simulink model "Backup_of_FOC_Simulate"  (R2016b)
settings: Solver=ode1  StartTime=0.0  StopTime=20  FixedStep=1e-5  RelTol=1e-3  EnableMultiTasking=on
undefined symbols (not defined in the file): sigbuilder_block
libraries: simulink x9, powerlib_meascontrol x4, powerlib x4
settings Model: ExtModeTrigDuration=8  Creator=tiend  LastModifiedBy=tiend

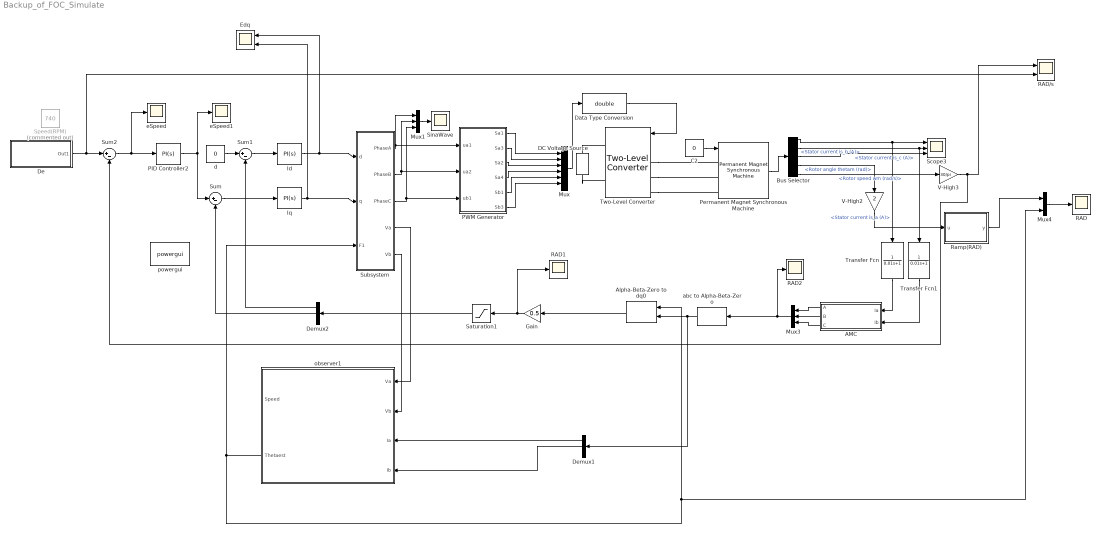
== system Backup_of_FOC_Simulate ==
  AMC : Subsystem
  Alpha-Beta-Zero to dq0 : powerlib_meascontrol/Transformations/Alpha-Beta-Zero to dq0  Alignment=Aligned with phase A axis
  Bus Selector : BusSelector  OutputSignals=Stator current is_a (A),Stator current is_b (A),Stator current is_c (A),Rotor angle thetam (rad),Rotor speed wm (rad/s)
  C2 : Constant  Value=0
  DC Voltage Source : powerlib/Electrical Sources/DC Voltage Source  Amplitude=300  Measurements=Voltage
  Data Type Conversion : DataTypeConversion  OutDataTypeStr=double
  De : Subsystem
  Demux1 : Demux  Outputs=3
  Demux2 : Demux  Outputs=3
  Edq : Scope  NumInputPorts=2
  Gain : Gain  Gain=0.5
  Id : simulink/Continuous/PID Controller  Controller=PI  TimeDomain=Continuous-time  SampleTime=-1  IntegratorMethod=Forward Euler  FilterMethod=Forward Euler  Form=Parallel  UseFilter=on  ControllerParametersSource=internal  P=0.5  I=0.5  D=0  N=100  InitialConditionSource=internal  InitialConditionForIntegrator=0  InitialConditionForFilter=0  ExternalReset=none  LimitOutput=off  UpperSaturationLimit=inf  LowerSaturationLimit=-inf  LinearizeAsGain=on  AntiWindupMode=none  Kb=1  TrackingMode=off  Kt=1  PParamMin=[]  PParamMax=[]  IParamMin=[]  IParamMax=[]  DParamMin=[]  DParamMax=[]  NParamMin=[]  NParamMax=[]  KbParamMin=[]  KbParamMax=[]  KtParamMin=[]  KtParamMax=[]  POutMin=[]  POutMax=[]  IOutMin=[]  IOutMax=[]  DOutMin=[]  DOutMax=[]  NOutMin=[]  NOutMax=[]  KbOutMin=[]  KbOutMax=[]  KtOutMin=[]  KtOutMax=[]  IntegratorOutMin=[]  IntegratorOutMax=[]  FilterOutMin=[]  FilterOutMax=[]  SumOutMin=[]  SumOutMax=[]  SumI1OutMin=[]  SumI1OutMax=[]  SumI2OutMin=[]  SumI2OutMax=[]  SumI3OutMin=[]  SumI3OutMax=[]  SumDOutMin=[]  SumDOutMax=[]  SaturationOutMin=[]  SaturationOutMax=[]  IntegratorContinuousStateAttributes=''  IntegratorStateMustResolveToSignalObject=off  IntegratorRTWStateStorageClass=Auto  FilterContinuousStateAttributes=''  FilterStateMustResolveToSignalObject=off  FilterRTWStateStorageClass=Auto  DifferentiatorICPrevScaledInput=0  DifferentiatorOutMin=[]  DifferentiatorOutMax=[]
  Iq : simulink/Continuous/PID Controller  Controller=PI  TimeDomain=Continuous-time  SampleTime=-1  IntegratorMethod=Forward Euler  FilterMethod=Forward Euler  Form=Parallel  UseFilter=on  ControllerParametersSource=internal  P=0.7  I=0.9  D=0  N=100  InitialConditionSource=internal  InitialConditionForIntegrator=0  InitialConditionForFilter=0  ExternalReset=none  LimitOutput=off  UpperSaturationLimit=inf  LowerSaturationLimit=-inf  LinearizeAsGain=on  AntiWindupMode=none  Kb=1  TrackingMode=off  Kt=1  PParamMin=[]  PParamMax=[]  IParamMin=[]  IParamMax=[]  DParamMin=[]  DParamMax=[]  NParamMin=[]  NParamMax=[]  KbParamMin=[]  KbParamMax=[]  KtParamMin=[]  KtParamMax=[]  POutMin=[]  POutMax=[]  IOutMin=[]  IOutMax=[]  DOutMin=[]  DOutMax=[]  NOutMin=[]  NOutMax=[]  KbOutMin=[]  KbOutMax=[]  KtOutMin=[]  KtOutMax=[]  IntegratorOutMin=[]  IntegratorOutMax=[]  FilterOutMin=[]  FilterOutMax=[]  SumOutMin=[]  SumOutMax=[]  SumI1OutMin=[]  SumI1OutMax=[]  SumI2OutMin=[]  SumI2OutMax=[]  SumI3OutMin=[]  SumI3OutMax=[]  SumDOutMin=[]  SumDOutMax=[]  SaturationOutMin=[]  SaturationOutMax=[]  IntegratorContinuousStateAttributes=''  IntegratorStateMustResolveToSignalObject=off  IntegratorRTWStateStorageClass=Auto  FilterContinuousStateAttributes=''  FilterStateMustResolveToSignalObject=off  FilterRTWStateStorageClass=Auto  DifferentiatorICPrevScaledInput=0  DifferentiatorOutMin=[]  DifferentiatorOutMax=[]
  Mux : Mux  Inputs=6
  Mux1 : Mux  Inputs=3
  Mux3 : Mux  Inputs=3
  Mux4 : Mux  Inputs=2
  PID Controller2 : simulink/Continuous/PID Controller  Controller=PI  TimeDomain=Continuous-time  SampleTime=-1  IntegratorMethod=Forward Euler  FilterMethod=Forward Euler  Form=Parallel  UseFilter=on  ControllerParametersSource=internal  P=1/50  I=0.01  D=0  N=100  InitialConditionSource=internal  InitialConditionForIntegrator=0  InitialConditionForFilter=0  ExternalReset=none  LimitOutput=off  UpperSaturationLimit=1  LowerSaturationLimit=-0.1  LinearizeAsGain=on  AntiWindupMode=none  Kb=1  TrackingMode=off  Kt=1  PParamMin=[]  PParamMax=[]  IParamMin=[]  IParamMax=[]  DParamMin=[]  DParamMax=[]  NParamMin=[]  NParamMax=[]  KbParamMin=[]  KbParamMax=[]  KtParamMin=[]  KtParamMax=[]  POutMin=[]  POutMax=[]  IOutMin=[]  IOutMax=[]  DOutMin=[]  DOutMax=[]  NOutMin=[]  NOutMax=[]  KbOutMin=[]  KbOutMax=[]  KtOutMin=[]  KtOutMax=[]  IntegratorOutMin=[]  IntegratorOutMax=[]  FilterOutMin=[]  FilterOutMax=[]  SumOutMin=[]  SumOutMax=[]  SumI1OutMin=[]  SumI1OutMax=[]  SumI2OutMin=[]  SumI2OutMax=[]  SumI3OutMin=[]  SumI3OutMax=[]  SumDOutMin=[]  SumDOutMax=[]  SaturationOutMin=[]  SaturationOutMax=[]  IntegratorContinuousStateAttributes=''  IntegratorStateMustResolveToSignalObject=off  IntegratorRTWStateStorageClass=Auto  FilterContinuousStateAttributes=''  FilterStateMustResolveToSignalObject=off  FilterRTWStateStorageClass=Auto  DifferentiatorICPrevScaledInput=0  DifferentiatorOutMin=[]  DifferentiatorOutMax=[]
  PWM Generator : Subsystem
  Permanent Magnet Synchronous Machine : powerlib/Machines/Permanent Magnet Synchronous Machine  NbPhases=3  FluxDistribution=Sinusoidal  RotorType=Round  MechanicalLoad=Torque Tm  PresetModel="01:  0.8 Nm 300 Vdc 3000 RPM - 0.8 Nm"  ShowDetailedParameters=on  MeasurementBus=off  Resistance=18.7  Inductance=8.5e-3  dqInductances=[8.5e-3,8.5e-3]  La=0.02682  MachineConstant=Flux linkage established by magnets (V.s)  Flux=0.1717  VoltageCst=62.2859  TorqueCst=0.5151  Flat=120  Mechanical=[2.26e-05 1.349e-05 2 0]  PolePairs=2  InitialConditions=[0,30, 0,0]  InitialConditions5ph=[0 0 0 0 0 0]  TsPowergui=0  TsBlock=-1  RefAngle=Aligned with phase A axis (original Park)
  RAD : Scope
  RAD/s : Scope  NumInputPorts=2
  RAD1 : Scope
  RAD2 : Scope
  Ramp(RAD) : MATLAB Function  TreatAsAtomicUnit=on
  Saturation1 : Saturate  UpperLimit=1  LowerLimit=-1
  Scope3 : Scope  NumInputPorts=3
  SinaWave : Scope
  Speed(RPM) : Constant  Commented=on  Value=740
  Subsystem : Subsystem
  Sum : Sum  Inputs=|+-
  Sum1 : Sum  Inputs=|+-
  Sum2 : Sum  Inputs=|+-
  Transfer Fcn : TransferFcn  Denominator=[0.01 1]
  Transfer Fcn1 : TransferFcn  Denominator=[0.01 1]
  Two-Level Converter : powerlib/Power Electronics/Two-Level Converter  ModelType=Switching devices  Ron=1e-3  Rs=1e6  Cs=inf  Vforward=[0,0]  Ron_Diode=1e-3  Rs_Diode=1e6  Cs_Diode=inf  Vf_Diode=1e-3  Rs_CurrentSource=inf
  V-High2 : Gain  Gain=2
  V-High3 : Gain  Gain=30/pi
  abc to Alpha-Beta-Zero : powerlib_meascontrol/Transformations/abc to Alpha-Beta-Zero
  d : Constant  Value=0
  eSpeed : Scope
  eSpeed1 : Scope
  observer1 : Subsystem  mask{R=0.0485, L=0.000395, Pva=20, Iva=0.1, Pvb=20, Ivb=0.1, K1=10, K2=5}
  powergui : powerlib/powergui  Priority=1  SimulationMode=Discrete  SolverType=Tustin/Backward Euler (TBE)  SampleTime=1e-5  frequency=60  SPID=off  DisableSnubberDevices=off  DisableRonSwitches=off  DisableVfSwitches=off  SwTol=0  DisplayEquations=off  Interpol=off  ExternalGateDelay=off  methode=off  Ts=10  FunctionMessages=off  echomessages=off  HookPort=off  EnableUseOfTLC=off  x0status=blocks  frequencyindice=0  Pbase=100e6  ErrMax=1e-4  Iterations=50  UnitsV=kV  UnitsW=MW  buscounter=0  RestoreLinks=warning  ResistiveCurrentMeasurement=off  Frange=[0:2:500]  Ylog=off  Xlog=on  ShowGrid=off  save=off  variable=ZData  structure=0  ZoomFFT=off  StartTime=0.0  cycles=1  DisplayStyle=1  fundamental=60  FreqAxis=off  MaxFrequency=1000  frequencyindicesteady=1  RmsSteady=1  display=off
  wires:
  Subsystem/3(PhaseC) -> PWM Generator/3(ub1), Mux1/3
  Subsystem/2(PhaseB) -> PWM Generator/2(ua2), Mux1/2
  PWM Generator/3(Sa2) -> Mux/3
  PWM Generator/4(Sa4) -> Mux/4
  PWM Generator/2(Sa3) -> Mux/2
  PWM Generator/5(Sb1) -> Mux/5
  PWM Generator/1(Sa1) -> Mux/1
  PWM Generator/6(Sb3) -> Mux/6
  C2/1 -> Permanent Magnet Synchronous Machine/1
  Mux/1 -> Data Type Conversion/1
  Data Type Conversion/1 -> Two-Level Converter/1
  Permanent Magnet Synchronous Machine/1 -> Bus Selector/1
  Mux1/1 -> SinaWave/1
  Subsystem/1(PhaseA) -> PWM Generator/1(ua1), Mux1/1
  Bus Selector/1 -> Scope3/1, Transfer Fcn/1  "<Stator current is_a (A)>"
  Bus Selector/2 -> Transfer Fcn1/1, Scope3/2  "<Stator current is_b (A)>"
  Bus Selector/3 -> Scope3/3  "<Stator current is_c (A)>"
  Bus Selector/4 -> V-High2/1  "<Rotor angle thetam (rad)>"
  AMC/3(C) -> Mux3/3
  AMC/2(B) -> Mux3/2
  AMC/1(A) -> Mux3/1
  Mux3/1 -> abc to Alpha-Beta-Zero/1, RAD2/1
  V-High2/1 -> Ramp(RAD)/1(u)
  Ramp(RAD)/1(y) -> Mux4/1
  Mux4/1 -> RAD/1
  Bus Selector/5 -> V-High3/1  "<Rotor speed wm (rad/s)>"
  Gain/1 -> Saturation1/1, RAD1/1
  d/1 -> Sum1/1
  Sum1/1 -> Id/1
  Id/1 -> Subsystem/1(d), Edq/1
  Sum2/1 -> PID Controller2/1, eSpeed/1
  PID Controller2/1 -> Sum/1, eSpeed1/1
  Saturation1/1 -> Demux2/1
  Demux2/1 -> Sum1/2
  De/1(Out1) -> RAD/s/2, Sum2/1
  Sum/1 -> Iq/1
  Demux2/2 -> Sum/2
  Iq/1 -> Subsystem/2(q), Edq/2
  Subsystem/5(Vb) -> observer1/2(Vb)
  Subsystem/4(Va) -> observer1/1(Va)
  observer1/2(Thetaest) -> Subsystem/3(F1), Alpha-Beta-Zero to dq0/2, Mux4/2
  abc to Alpha-Beta-Zero/1 -> Demux1/1, Alpha-Beta-Zero to dq0/1
  Alpha-Beta-Zero to dq0/1 -> Gain/1
  Demux1/1 -> observer1/3(Ia)
  Demux1/2 -> observer1/4(Ib)
  Transfer Fcn1/1 -> AMC/2(Ib)
  Transfer Fcn/1 -> AMC/1(Ia)
  V-High3/1 -> Sum2/2, RAD/s/1
  connections:
  Two-Level Converter/LConn1 -- Permanent Magnet Synchronous Machine/LConn1
  Two-Level Converter/LConn2 -- Permanent Magnet Synchronous Machine/LConn2
  Two-Level Converter/LConn3 -- Permanent Magnet Synchronous Machine/LConn3
  DC Voltage Source/RConn1 -- Two-Level Converter/RConn1
  DC Voltage Source/LConn1 -- Two-Level Converter/RConn2

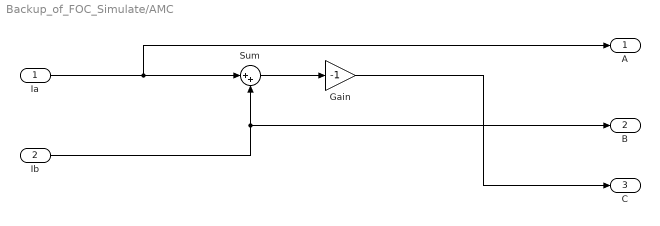
== system Backup_of_FOC_Simulate/AMC ==
  Ia : Inport
  Ib : Inport  Port=2
  Gain : Gain  Gain=-1
  Sum : Sum  Inputs=|++
  A : Outport
  B : Outport  Port=2
  C : Outport  Port=3
  wires:
  Sum/1 -> Gain/1
  Ia/1 -> A/1, Sum/1
  Ib/1 -> B/1, Sum/2
  Gain/1 -> C/1

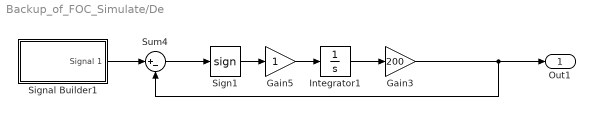
== system Backup_of_FOC_Simulate/De ==
  Gain3 : Gain  Gain=200
  Gain5 : Gain
  Integrator1 : Integrator
  Sign1 : Signum  ZeroCross=off
  Signal Builder1 : Subsystem  Tag=STV Subsys  LoadFcn=sigbuilder_block('load');  StartFcn=sigbuilder_block('start');  StopFcn=sigbuilder_block('stop');  ClipboardFcn=sigbuilder_block('clipboard');  mask(Sigbuilder block){tuvar=[0:10]}
      mask help: Simulink:masks:SigbuilderBlock_MD
      mask init:
      | if ~strcmp(get_param(bdroot(gcbh),'SimulationStatus'),'stopped') tuvar = sigbuilder_block('maskInit'); end
      settings: CopyFcn=sigbuilder_block('copy');  DeleteFcn=sigbuilder_block('delete');  ModelCloseFcn=sigbuilder_block('modelClose');  PreSaveFcn=sigbuilder_block('preSave');  PauseFcn=sigbuilder_block('pause');  ContinueFcn=sigbuilder_block('continue');  NameChangeFcn=sigbuilder_block('namechange');  OpenFcn=sigbuilder_block('open',[437.25 153 550.5 359.25 ]);  CloseFcn=sigbuilder_block('close');
      mask Display: plot(0, 0, 100, 100,[2, 2, 32, 32, 2], [68, 8, 8, 68, 68],[32, 2], [38, 38], [32, 19, 2],[53, 60, 44], [32, 17, 17, 2],[16, 16, 31, 31]);txt = getActiveGroup(gcbh);text(2, 100, txt,'verticalAlignment', 'top');
  Sum4 : Sum  Inputs=|+-
  Out1 : Outport
  wires:
  Signal Builder1/1(Signal 1) -> Sum4/1
  Integrator1/1 -> Gain3/1
  Sum4/1 -> Sign1/1
  Sign1/1 -> Gain5/1
  Gain5/1 -> Integrator1/1
  Gain3/1 -> Out1/1, Sum4/2

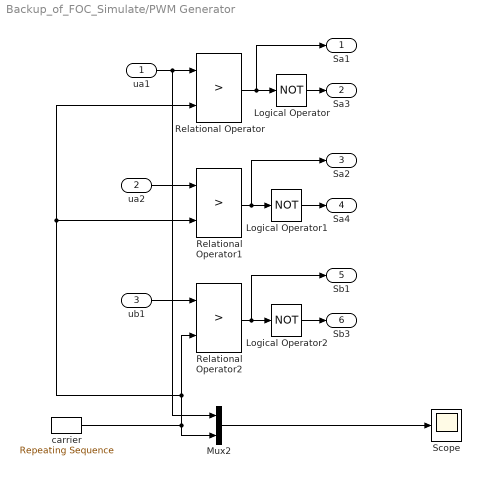
== system Backup_of_FOC_Simulate/PWM Generator ==
  ua1 : Inport
  ua2 : Inport  Port=2
  ub1 : Inport  Port=3
  Logical Operator : Logic  Operator=NOT  AllPortsSameDT=off  OutDataTypeStr=boolean
  Logical Operator1 : Logic  Operator=NOT  AllPortsSameDT=off  OutDataTypeStr=boolean
  Logical Operator2 : Logic  Operator=NOT  AllPortsSameDT=off  OutDataTypeStr=boolean
  Mux2 : Mux  Inputs=2
  Relational Operator : RelationalOperator  Operator=>  OutDataTypeStr=boolean  RndMeth=Nearest
  Relational Operator1 : RelationalOperator  Operator=>  OutDataTypeStr=boolean  RndMeth=Nearest
  Relational Operator2 : RelationalOperator  Operator=>  OutDataTypeStr=boolean  RndMeth=Nearest
  Scope : Scope
  carrier : simulink/Sources/Repeating Sequence  rep_seq_t=[0 1/20000 1/10000]  rep_seq_y=[0 1 0]
  Sa1 : Outport
  Sa3 : Outport  Port=2
  Sa2 : Outport  Port=3
  Sa4 : Outport  Port=4
  Sb1 : Outport  Port=5
  Sb3 : Outport  Port=6
  wires:
  Logical Operator2/1 -> Sb3/1
  Logical Operator1/1 -> Sa4/1
  ub1/1 -> Relational Operator2/1
  ua2/1 -> Relational Operator1/1
  Relational Operator2/1 -> Sb1/1, Logical Operator2/1
  Relational Operator1/1 -> Sa2/1, Logical Operator1/1
  ua1/1 -> Mux2/1, Relational Operator/1
  Relational Operator/1 -> Logical Operator/1, Sa1/1
  Logical Operator/1 -> Sa3/1
  carrier/1 -> Mux2/2, Relational Operator/2, Relational Operator1/2, Relational Operator2/2
  Mux2/1 -> Scope/1

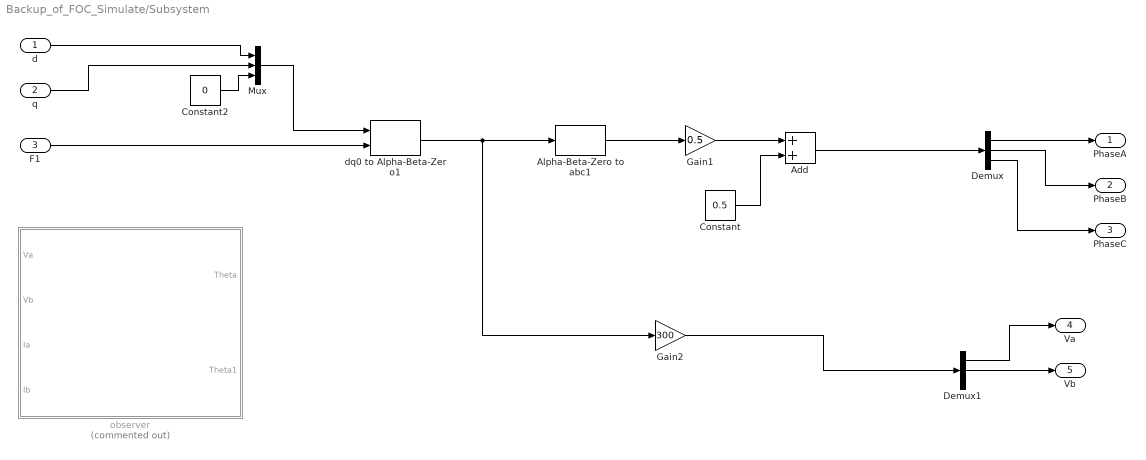
== system Backup_of_FOC_Simulate/Subsystem ==
  d : Inport
  q : Inport  Port=2
  F1 : Inport  Port=3
  Add : Sum
  Alpha-Beta-Zero to abc1 : powerlib_meascontrol/Transformations/Alpha-Beta-Zero to abc
  Constant : Constant  Value=0.5  SampleTime=-1
  Constant2 : Constant  Value=0  SampleTime=-1
  Demux : Demux  Outputs=3
  Demux1 : Demux  Outputs=3
  Gain1 : Gain  Gain=0.5
  Gain2 : Gain  Gain=300
  Mux : Mux  Inputs=3
  dq0 to Alpha-Beta-Zero1 : powerlib_meascontrol/Transformations/dq0 to Alpha-Beta-Zero  Alignment=Aligned with phase A axis
  observer : Subsystem  Commented=on  mask{R=0.0485, L=0.000395, Pva=17, Iva=0.1, Pvb=17, Ivb=0.1, K1=10, K2=5}
  PhaseA : Outport
  PhaseB : Outport  Port=2
  PhaseC : Outport  Port=3
  Va : Outport  Port=4
  Vb : Outport  Port=5
  wires:
  Constant/1 -> Add/2
  Alpha-Beta-Zero to abc1/1 -> Gain1/1
  Demux/1 -> PhaseA/1
  Demux/2 -> PhaseB/1
  Demux/3 -> PhaseC/1
  Mux/1 -> dq0 to Alpha-Beta-Zero1/1
  Add/1 -> Demux/1
  Constant2/1 -> Mux/3
  d/1 -> Mux/1
  Gain1/1 -> Add/1
  F1/1 -> dq0 to Alpha-Beta-Zero1/2
  q/1 -> Mux/2
  dq0 to Alpha-Beta-Zero1/1 -> Gain2/1, Alpha-Beta-Zero to abc1/1
  Demux1/1 -> Va/1
  Demux1/2 -> Vb/1
  Gain2/1 -> Demux1/1

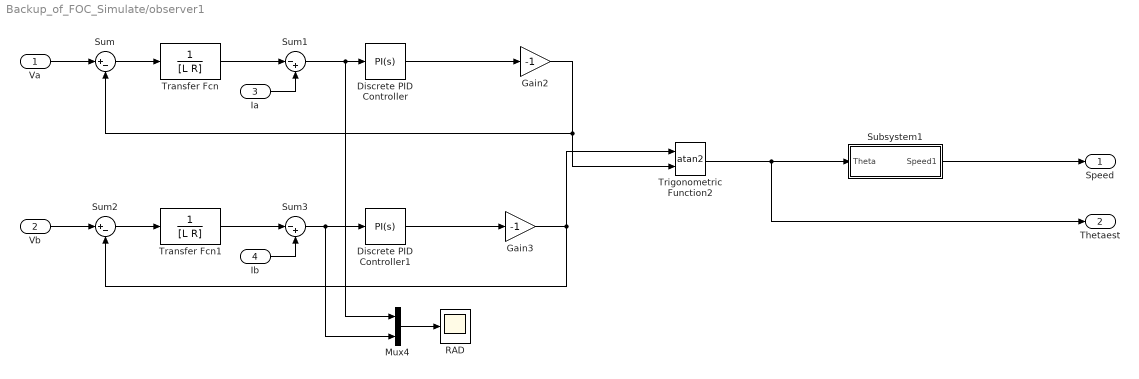
== system Backup_of_FOC_Simulate/observer1 ==
  Va : Inport
  Vb : Inport  Port=2
  Ia : Inport  Port=3
  Ib : Inport  Port=4
  Discrete PID Controller : simulink/Continuous/PID Controller  Controller=PI  TimeDomain=Continuous-time  SampleTime=-1  IntegratorMethod=Forward Euler  FilterMethod=Forward Euler  Form=Parallel  UseFilter=on  ControllerParametersSource=internal  P=Pva  I=Iva  D=0  N=100  InitialConditionSource=internal  InitialConditionForIntegrator=0  InitialConditionForFilter=0  ExternalReset=none  LimitOutput=off  UpperSaturationLimit=inf  LowerSaturationLimit=-inf  LinearizeAsGain=off  AntiWindupMode=none  Kb=1  TrackingMode=off  Kt=1  PParamMin=[]  PParamMax=[]  IParamMin=[]  IParamMax=[]  DParamMin=[]  DParamMax=[]  NParamMin=[]  NParamMax=[]  KbParamMin=[]  KbParamMax=[]  KtParamMin=[]  KtParamMax=[]  POutMin=[]  POutMax=[]  IOutMin=[]  IOutMax=[]  DOutMin=[]  DOutMax=[]  NOutMin=[]  NOutMax=[]  KbOutMin=[]  KbOutMax=[]  KtOutMin=[]  KtOutMax=[]  IntegratorOutMin=[]  IntegratorOutMax=[]  FilterOutMin=[]  FilterOutMax=[]  SumOutMin=[]  SumOutMax=[]  SumI1OutMin=[]  SumI1OutMax=[]  SumI2OutMin=[]  SumI2OutMax=[]  SumI3OutMin=[]  SumI3OutMax=[]  SumDOutMin=[]  SumDOutMax=[]  SaturationOutMin=[]  SaturationOutMax=[]  IntegratorContinuousStateAttributes=''  IntegratorStateMustResolveToSignalObject=off  IntegratorRTWStateStorageClass=Auto  FilterContinuousStateAttributes=''  FilterStateMustResolveToSignalObject=off  FilterRTWStateStorageClass=Auto  DifferentiatorICPrevScaledInput=0  DifferentiatorOutMin=[]  DifferentiatorOutMax=[]
  Discrete PID Controller1 : simulink/Continuous/PID Controller  Controller=PI  TimeDomain=Continuous-time  SampleTime=-1  IntegratorMethod=Forward Euler  FilterMethod=Forward Euler  Form=Parallel  UseFilter=on  ControllerParametersSource=internal  P=Pvb  I=Ivb  D=0  N=100  InitialConditionSource=internal  InitialConditionForIntegrator=0  InitialConditionForFilter=0  ExternalReset=none  LimitOutput=off  UpperSaturationLimit=inf  LowerSaturationLimit=-inf  LinearizeAsGain=off  AntiWindupMode=none  Kb=1  TrackingMode=off  Kt=1  PParamMin=[]  PParamMax=[]  IParamMin=[]  IParamMax=[]  DParamMin=[]  DParamMax=[]  NParamMin=[]  NParamMax=[]  KbParamMin=[]  KbParamMax=[]  KtParamMin=[]  KtParamMax=[]  POutMin=[]  POutMax=[]  IOutMin=[]  IOutMax=[]  DOutMin=[]  DOutMax=[]  NOutMin=[]  NOutMax=[]  KbOutMin=[]  KbOutMax=[]  KtOutMin=[]  KtOutMax=[]  IntegratorOutMin=[]  IntegratorOutMax=[]  FilterOutMin=[]  FilterOutMax=[]  SumOutMin=[]  SumOutMax=[]  SumI1OutMin=[]  SumI1OutMax=[]  SumI2OutMin=[]  SumI2OutMax=[]  SumI3OutMin=[]  SumI3OutMax=[]  SumDOutMin=[]  SumDOutMax=[]  SaturationOutMin=[]  SaturationOutMax=[]  IntegratorContinuousStateAttributes=''  IntegratorStateMustResolveToSignalObject=off  IntegratorRTWStateStorageClass=Auto  FilterContinuousStateAttributes=''  FilterStateMustResolveToSignalObject=off  FilterRTWStateStorageClass=Auto  DifferentiatorICPrevScaledInput=0  DifferentiatorOutMin=[]  DifferentiatorOutMax=[]
  Gain2 : Gain  Gain=-1
  Gain3 : Gain  Gain=-1
  Mux4 : Mux  Inputs=2
  RAD : Scope
  Subsystem1 : Subsystem
  Sum : Sum  Inputs=|+-
  Sum1 : Sum  Inputs=|-+
  Sum2 : Sum  Inputs=|+-
  Sum3 : Sum  Inputs=|-+
  Transfer Fcn : TransferFcn  Denominator=[L R]
  Transfer Fcn1 : TransferFcn  Denominator=[L R]
  Trigonometric Function2 : Trigonometry  Operator=atan2
  Speed : Outport
  Thetaest : Outport  Port=2
  wires:
  Va/1 -> Sum/1
  Sum/1 -> Transfer Fcn/1
  Vb/1 -> Sum2/1
  Sum2/1 -> Transfer Fcn1/1
  Transfer Fcn/1 -> Sum1/1
  Sum1/1 -> Mux4/1, Discrete PID Controller/1
  Transfer Fcn1/1 -> Sum3/1
  Sum3/1 -> Mux4/2, Discrete PID Controller1/1
  Ia/1 -> Sum1/2
  Ib/1 -> Sum3/2
  Discrete PID Controller1/1 -> Gain3/1
  Gain3/1 -> Sum2/2, Trigonometric Function2/1
  Discrete PID Controller/1 -> Gain2/1
  Mux4/1 -> RAD/1
  Gain2/1 -> Trigonometric Function2/2, Sum/2
  Trigonometric Function2/1 -> Thetaest/1, Subsystem1/1(Theta)
  Subsystem1/1(Speed1) -> Speed/1

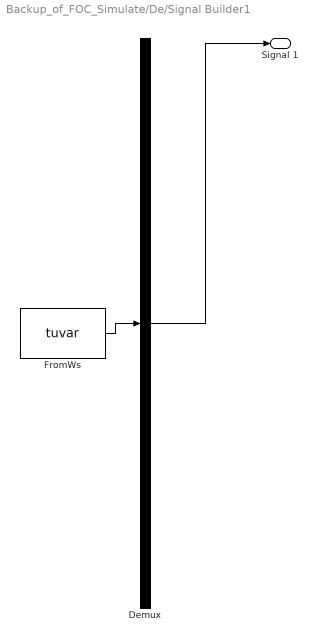
== system Backup_of_FOC_Simulate/De/Signal Builder1 ==
  Demux : Demux  Tag=STV Demux  Outputs=1
  FromWs : FromWorkspace  Tag=STV FromWs  VariableName=tuvar  SampleTime=0
      SigBuilderData=|
      | common.afterFinalStr = 'Extrapolate'
      | common.sampleTime = 0
      | dataSet.timeRange = [0 100]
      | dataSet.name = 'Group 1'
      | sbobj.Groups.Name = 'Group 1'
      | sbobj.Groups.Signals.Name = 'Signal 1'
      | sbobj.Groups.Signals.XData = [0 1 1 7 7 15 15 40 40 60 60 100]
      | sbobj.Groups.Signals.YData = [0 0 500 500 1500 1500 3000 3000 400 400 0 0]
      | sbobj.Groups.TimeRange = [0 100]
  Signal 1 : Outport  Tag=STV Outport
  wires:
  Demux/1 -> Signal 1/1
  FromWs/1 -> Demux/1

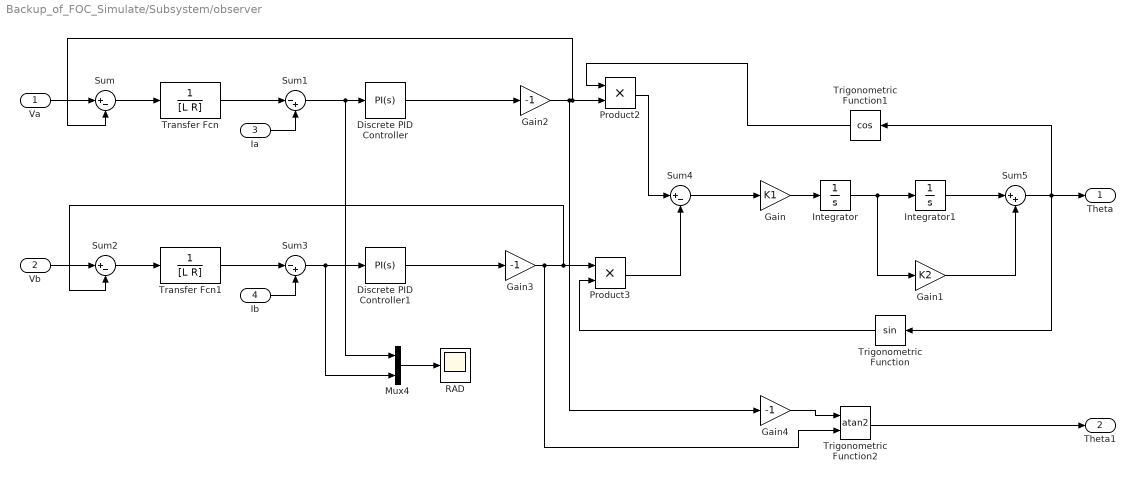
== system Backup_of_FOC_Simulate/Subsystem/observer ==
  Va : Inport
  Vb : Inport  Port=2
  Ia : Inport  Port=3
  Ib : Inport  Port=4
  Discrete PID Controller : simulink/Continuous/PID Controller  Controller=PI  TimeDomain=Continuous-time  SampleTime=-1  IntegratorMethod=Forward Euler  FilterMethod=Forward Euler  Form=Parallel  UseFilter=on  ControllerParametersSource=internal  P=Pva  I=Iva  D=0  N=100  InitialConditionSource=internal  InitialConditionForIntegrator=0  InitialConditionForFilter=0  ExternalReset=none  LimitOutput=off  UpperSaturationLimit=inf  LowerSaturationLimit=-inf  LinearizeAsGain=off  AntiWindupMode=none  Kb=1  TrackingMode=off  Kt=1  PParamMin=[]  PParamMax=[]  IParamMin=[]  IParamMax=[]  DParamMin=[]  DParamMax=[]  NParamMin=[]  NParamMax=[]  KbParamMin=[]  KbParamMax=[]  KtParamMin=[]  KtParamMax=[]  POutMin=[]  POutMax=[]  IOutMin=[]  IOutMax=[]  DOutMin=[]  DOutMax=[]  NOutMin=[]  NOutMax=[]  KbOutMin=[]  KbOutMax=[]  KtOutMin=[]  KtOutMax=[]  IntegratorOutMin=[]  IntegratorOutMax=[]  FilterOutMin=[]  FilterOutMax=[]  SumOutMin=[]  SumOutMax=[]  SumI1OutMin=[]  SumI1OutMax=[]  SumI2OutMin=[]  SumI2OutMax=[]  SumI3OutMin=[]  SumI3OutMax=[]  SumDOutMin=[]  SumDOutMax=[]  SaturationOutMin=[]  SaturationOutMax=[]  IntegratorContinuousStateAttributes=''  IntegratorStateMustResolveToSignalObject=off  IntegratorRTWStateStorageClass=Auto  FilterContinuousStateAttributes=''  FilterStateMustResolveToSignalObject=off  FilterRTWStateStorageClass=Auto  DifferentiatorICPrevScaledInput=0  DifferentiatorOutMin=[]  DifferentiatorOutMax=[]
  Discrete PID Controller1 : simulink/Continuous/PID Controller  Controller=PI  TimeDomain=Continuous-time  SampleTime=-1  IntegratorMethod=Forward Euler  FilterMethod=Forward Euler  Form=Parallel  UseFilter=on  ControllerParametersSource=internal  P=Pvb  I=Ivb  D=0  N=100  InitialConditionSource=internal  InitialConditionForIntegrator=0  InitialConditionForFilter=0  ExternalReset=none  LimitOutput=off  UpperSaturationLimit=inf  LowerSaturationLimit=-inf  LinearizeAsGain=off  AntiWindupMode=none  Kb=1  TrackingMode=off  Kt=1  PParamMin=[]  PParamMax=[]  IParamMin=[]  IParamMax=[]  DParamMin=[]  DParamMax=[]  NParamMin=[]  NParamMax=[]  KbParamMin=[]  KbParamMax=[]  KtParamMin=[]  KtParamMax=[]  POutMin=[]  POutMax=[]  IOutMin=[]  IOutMax=[]  DOutMin=[]  DOutMax=[]  NOutMin=[]  NOutMax=[]  KbOutMin=[]  KbOutMax=[]  KtOutMin=[]  KtOutMax=[]  IntegratorOutMin=[]  IntegratorOutMax=[]  FilterOutMin=[]  FilterOutMax=[]  SumOutMin=[]  SumOutMax=[]  SumI1OutMin=[]  SumI1OutMax=[]  SumI2OutMin=[]  SumI2OutMax=[]  SumI3OutMin=[]  SumI3OutMax=[]  SumDOutMin=[]  SumDOutMax=[]  SaturationOutMin=[]  SaturationOutMax=[]  IntegratorContinuousStateAttributes=''  IntegratorStateMustResolveToSignalObject=off  IntegratorRTWStateStorageClass=Auto  FilterContinuousStateAttributes=''  FilterStateMustResolveToSignalObject=off  FilterRTWStateStorageClass=Auto  DifferentiatorICPrevScaledInput=0  DifferentiatorOutMin=[]  DifferentiatorOutMax=[]
  Gain : Gain  Gain=K1
  Gain1 : Gain  Gain=K2
  Gain2 : Gain  Gain=-1
  Gain3 : Gain  Gain=-1
  Gain4 : Gain  Gain=-1
  Integrator : Integrator
  Integrator1 : Integrator
  Mux4 : Mux  Inputs=2
  Product2 : Product
  Product3 : Product
  RAD : Scope
  Sum : Sum  Inputs=|+-
  Sum1 : Sum  Inputs=|-+
  Sum2 : Sum  Inputs=|+-
  Sum3 : Sum  Inputs=|-+
  Sum4 : Sum  Inputs=|+-
  Sum5 : Sum  Inputs=|++
  Transfer Fcn : TransferFcn  Denominator=[L R]
  Transfer Fcn1 : TransferFcn  Denominator=[L R]
  Trigonometric Function : Trigonometry
  Trigonometric Function1 : Trigonometry  Operator=cos
  Trigonometric Function2 : Trigonometry  Operator=atan2
  Theta : Outport
  Theta1 : Outport  Port=2
  wires:
  Va/1 -> Sum/1
  Sum/1 -> Transfer Fcn/1
  Vb/1 -> Sum2/1
  Sum2/1 -> Transfer Fcn1/1
  Transfer Fcn/1 -> Sum1/1
  Sum1/1 -> Mux4/1, Discrete PID Controller/1
  Transfer Fcn1/1 -> Sum3/1
  Sum3/1 -> Mux4/2, Discrete PID Controller1/1
  Ia/1 -> Sum1/2
  Ib/1 -> Sum3/2
  Discrete PID Controller1/1 -> Gain3/1
  Gain3/1 -> Trigonometric Function2/2, Product3/1, Sum2/2
  Product2/1 -> Sum4/1
  Product3/1 -> Sum4/2
  Sum4/1 -> Gain/1
  Gain/1 -> Integrator/1
  Integrator/1 -> Gain1/1, Integrator1/1
  Integrator1/1 -> Sum5/1
  Gain1/1 -> Sum5/2
  Sum5/1 -> Trigonometric Function1/1, Trigonometric Function/1, Theta/1
  Trigonometric Function1/1 -> Product2/1
  Trigonometric Function/1 -> Product3/2
  Discrete PID Controller/1 -> Gain2/1
  Mux4/1 -> RAD/1
  Gain2/1 -> Gain4/1, Sum/2, Product2/2
  Gain4/1 -> Trigonometric Function2/1
  Trigonometric Function2/1 -> Theta1/1

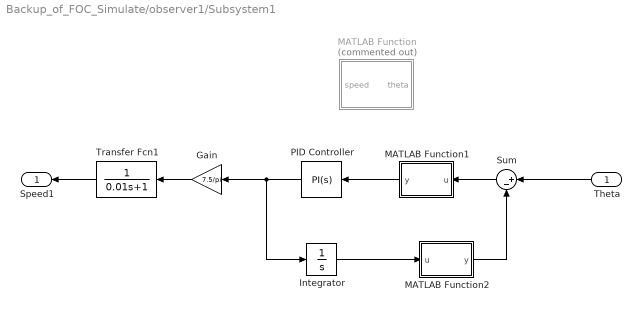
== system Backup_of_FOC_Simulate/observer1/Subsystem1 ==
  Theta : Inport
  Gain : Gain  Gain=7.5/pi
  Integrator : Integrator
  MATLAB Function : MATLAB Function  Commented=on  TreatAsAtomicUnit=on
  MATLAB Function1 : MATLAB Function  TreatAsAtomicUnit=on
  MATLAB Function2 : MATLAB Function  TreatAsAtomicUnit=on
  PID Controller : simulink/Continuous/PID Controller  Controller=PI  TimeDomain=Continuous-time  SampleTime=-1  IntegratorMethod=Forward Euler  FilterMethod=Forward Euler  Form=Parallel  UseFilter=on  ControllerParametersSource=internal  P=400  I=5  D=0  N=100  InitialConditionSource=internal  InitialConditionForIntegrator=0  InitialConditionForFilter=0  ExternalReset=none  LimitOutput=off  UpperSaturationLimit=inf  LowerSaturationLimit=-inf  LinearizeAsGain=on  AntiWindupMode=none  Kb=1  TrackingMode=off  Kt=1  PParamMin=[]  PParamMax=[]  IParamMin=[]  IParamMax=[]  DParamMin=[]  DParamMax=[]  NParamMin=[]  NParamMax=[]  KbParamMin=[]  KbParamMax=[]  KtParamMin=[]  KtParamMax=[]  POutMin=[]  POutMax=[]  IOutMin=[]  IOutMax=[]  DOutMin=[]  DOutMax=[]  NOutMin=[]  NOutMax=[]  KbOutMin=[]  KbOutMax=[]  KtOutMin=[]  KtOutMax=[]  IntegratorOutMin=[]  IntegratorOutMax=[]  FilterOutMin=[]  FilterOutMax=[]  SumOutMin=[]  SumOutMax=[]  SumI1OutMin=[]  SumI1OutMax=[]  SumI2OutMin=[]  SumI2OutMax=[]  SumI3OutMin=[]  SumI3OutMax=[]  SumDOutMin=[]  SumDOutMax=[]  SaturationOutMin=[]  SaturationOutMax=[]  IntegratorContinuousStateAttributes=''  IntegratorStateMustResolveToSignalObject=off  IntegratorRTWStateStorageClass=Auto  FilterContinuousStateAttributes=''  FilterStateMustResolveToSignalObject=off  FilterRTWStateStorageClass=Auto  DifferentiatorICPrevScaledInput=0  DifferentiatorOutMin=[]  DifferentiatorOutMax=[]
  Sum : Sum  Inputs=|+-
  Transfer Fcn1 : TransferFcn  Denominator=[0.01 1]
  Speed1 : Outport
  wires:
  PID Controller/1 -> Integrator/1, Gain/1
  Gain/1 -> Transfer Fcn1/1
  Sum/1 -> MATLAB Function1/1(u)
  Theta/1 -> Sum/1
  Integrator/1 -> MATLAB Function2/1(u)
  MATLAB Function1/1(y) -> PID Controller/1
  Transfer Fcn1/1 -> Speed1/1
  MATLAB Function2/1(y) -> Sum/2

== matlab function Backup_of_FOC_Simulate/Ramp(RAD) ==
  data: u input; y output
function y = fcn(u)
if u>=(2*pi)
    u=mod(u,2*pi);
end
y = u;

== matlab function Backup_of_FOC_Simulate/observer1/Subsystem1/MATLAB Function ==
  data: theta input; speed output
function speed = fcn(theta)
Kp = 0.1; Ki = 0.3; dt = 1e-5;
persistent pll_theta speed_pll
if isempty(pll_theta)
    pll_theta = 0;
    speed_pll = 0;
end
delta_theta = theta - pll_theta;
while(delta_theta >= pi) delta_theta = delta_theta-2*pi; end
while(delta_theta <= -pi) delta_theta = delta_theta + 2*pi; end
 pll_theta = pll_theta + (speed_pll + Kp*delta_theta)*dt;
 
while(pll_theta >= pi)
    pll_theta = pll_theta - 2*pi; 
end

while(pll_theta <= -pi) 
    pll_theta = pll_theta + 2*pi; 
end
 
speed_pll = speed_pll + Ki*delta_theta*dt;    
speed = speed_pll;

== matlab function Backup_of_FOC_Simulate/observer1/Subsystem1/MATLAB Function1 ==
  data: u input; y output
function y = fcn(u)
theta = u;
while(theta >= pi) theta = theta - 2*pi; end
while (theta <= -pi) theta = theta + 2*pi; end
y = theta;

== matlab function Backup_of_FOC_Simulate/observer1/Subsystem1/MATLAB Function2 ==
  data: u input; y output
function y = fcn(u)
theta = u;
while(theta >= pi) theta = theta - 2*pi; end
while (theta <= -pi) theta = theta + 2*pi; end
y = theta;
